simulink model "segmentCalcPos"  (R2019a)
settings: Solver=VariableStepAuto  StartTime=0  StopTime=inf  FixedStep=1e-3  MaxStep=1e-3  RelTol=1e-3
values from neighbouring files (symbols this model uses):
  apexVelocity = apexData.velocity(n,2)    [calcSegments.m]
  course = addRadius(course,max(vRLookUp(:,1)))    [calcggV.m]    (also in importCourse.m = addRadius(course))
  currentDistance = apexData.locs(n,1) - 1    [calcSegments.m]
  stoppingDistance = apexData.locs(n+1,1) - 1    [calcSegments.m]
undefined symbols (not defined in the file or in its folder): aeroMap, init
libraries: simulink x1
settings Model: Creator=Frieder Uerlings  LastModifiedBy=fried

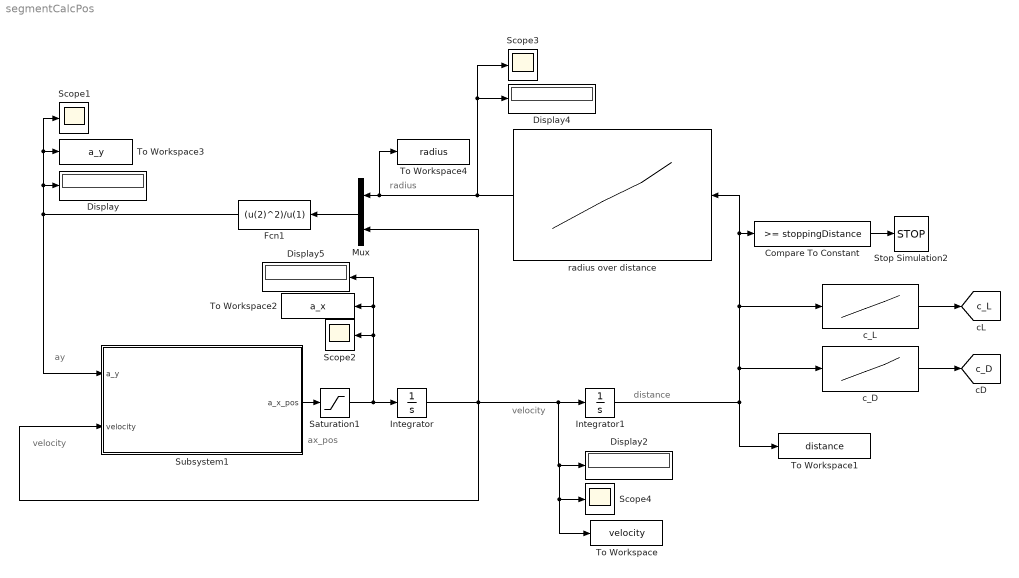
== system segmentCalcPos ==
  note: radius
  note: distance
  note: velocity
  note: velocity
  note: ay
  note: ax_pos
  Compare To Constant : simulink/Logic and Bit Operations/Compare To Constant  relop=>=  const=stoppingDistance  OutDataTypeStr=boolean
  Display{,2,4..5} (4 alike) : Display
  Fcn1 : Fcn  Expr=(u(2)^2)/u(1)
  Integrator : Integrator  InitialCondition=apexVelocity
  Integrator1 : Integrator  InitialCondition=currentDistance
  Mux : Mux  Inputs=2
  Saturation1 : Saturate  UpperLimit=inf  LowerLimit=0
  Scope{1..4} (4 alike) : Scope
  Stop Simulation2 : Stop
  Subsystem1 : Subsystem
  To Workspace : ToWorkspace  VariableName=velocity  SampleTime=-1
  To Workspace1 : ToWorkspace  VariableName=distance  SampleTime=-1
  To Workspace2 : ToWorkspace  VariableName=a_x  SampleTime=-1
  To Workspace3 : ToWorkspace  VariableName=a_y  SampleTime=-1
  To Workspace4 : ToWorkspace  VariableName=radius  SampleTime=-1
  "c_D " : Lookup_n-D  NumberOfTableDimensions=1  BreakpointsForDimension1=[0:init.ptDistance:(length(course)-1)*init.ptDistance]  Table=aeroMap(:,2)  InternalRulePriority=Speed  RndMeth=Simplest  InputSameDT=on
  c_L : Lookup_n-D  NumberOfTableDimensions=1  BreakpointsForDimension1=[0:init.ptDistance:(length(course)-1)*init.ptDistance]  Table=aeroMap(:,1)  InternalRulePriority=Speed  RndMeth=Simplest  InputSameDT=on
  radius over distance : Lookup_n-D  NumberOfTableDimensions=1  BreakpointsForDimension1=[0:init.ptDistance:(length(course)-1)*init.ptDistance]  Table=course(:,3)  InternalRulePriority=Speed  RndMeth=Simplest  InputSameDT=on
  tag scope: c_D=global, c_L=global
  wires:
  Integrator1/1 -> To Workspace1/1, "c_D "/1, c_L/1, Compare To Constant/1, radius over distance/1
  Subsystem1/1("a_x_pos ") -> Saturation1/1
  radius over distance/1 -> Scope3/1, Display4/1, To Workspace4/1, Mux/1
  Mux/1 -> Fcn1/1
  Compare To Constant/1 -> Stop Simulation2/1
  Integrator/1 -> Subsystem1/2("velocity "), Mux/2, To Workspace/1, Scope4/1, Display2/1, Integrator1/1
  Saturation1/1 -> Display5/1, To Workspace2/1, Scope2/1, Integrator/1
  Fcn1/1 -> Subsystem1/1("a_y "), Display/1, Scope1/1, To Workspace3/1
  "c_D "/1 -> [c_D]
  c_L/1 -> [c_L]

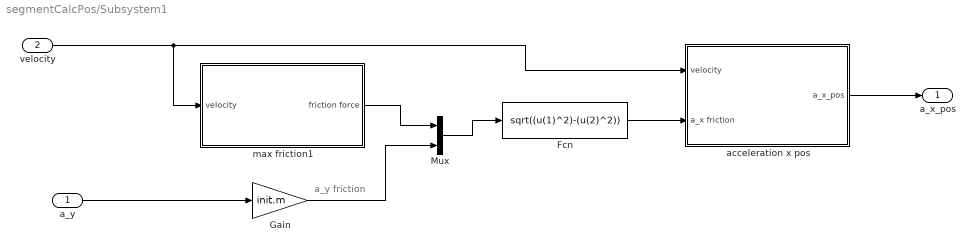
== system segmentCalcPos/Subsystem1 ==
  note: a_y friction
  "a_y " : Inport
  "velocity " : Inport  Port=2
  Fcn : Fcn  Expr=sqrt((u(1)^2)-(u(2)^2))
  Gain : Gain  Gain=init.m
  Mux : Mux  Inputs=2
  acceleration x pos : Subsystem
  max friction1 : Subsystem
  "a_x_pos " : Outport
  wires:
  "velocity "/1 -> acceleration x pos/1(velocity), max friction1/1(velocity)
  "a_y "/1 -> Gain/1
  Fcn/1 -> acceleration x pos/2(a_x friction)
  Mux/1 -> Fcn/1
  acceleration x pos/1("a_x_pos ") -> "a_x_pos "/1
  max friction1/1(friction force) -> Mux/1
  Gain/1 -> Mux/2

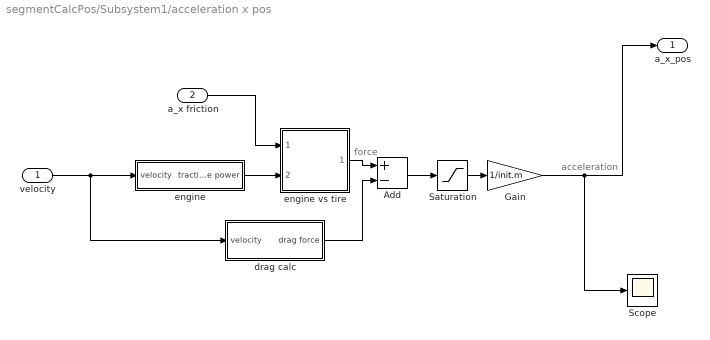
== system segmentCalcPos/Subsystem1/acceleration x pos ==
  note: force
  note: acceleration
  velocity : Inport
  a_x friction : Inport  Port=2
  Add : Sum  Inputs=+-
  Gain : Gain  Gain=1/init.m
  Saturation : Saturate  UpperLimit=inf  LowerLimit=0
  Scope : Scope
  drag calc : Subsystem
  engine : Subsystem
  engine vs tire : Subsystem
  "a_x_pos " : Outport
  wires:
  engine vs tire/1(acc force) -> Add/1
  Gain/1 -> "a_x_pos "/1, Scope/1
  Add/1 -> Saturation/1
  drag calc/1("drag force ") -> Add/2
  engine/1(tractive power) -> engine vs tire/2(tractive power)
  a_x friction/1 -> engine vs tire/1("a_x friction ")
  velocity/1 -> drag calc/1(velocity), engine/1(velocity)
  Saturation/1 -> Gain/1

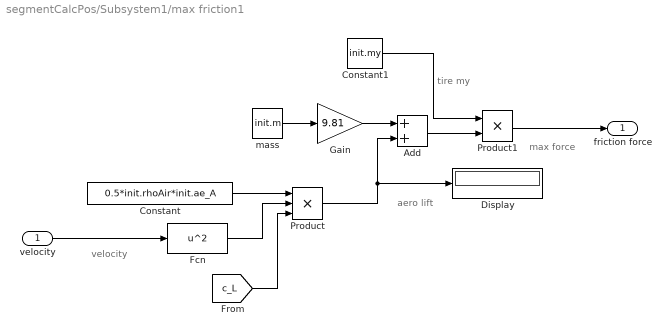
== system segmentCalcPos/Subsystem1/max friction1 ==
  note: velocity
  note: tire my
  note: aero lift
  note: max force
  velocity : Inport
  Add : Sum
  Constant : Constant  Value=0.5*init.rhoAir*init.ae_A
  Constant1 : Constant  Value=init.my
  Display : Display
  Fcn : Fcn  Expr=u^2
  Gain : Gain  Gain=9.81
  Product : Product  Inputs=3
  Product1 : Product
  "mass " : Constant  Value=init.m
  friction force : Outport
  wires:
  Product/1 -> Display/1, Add/2
  velocity/1 -> Fcn/1
  Constant1/1 -> Product1/1
  Gain/1 -> Add/1
  Product1/1 -> friction force/1
  Fcn/1 -> Product/2
  "mass "/1 -> Gain/1
  Add/1 -> Product1/2
  Constant/1 -> Product/1
  [c_L] -> Product/3

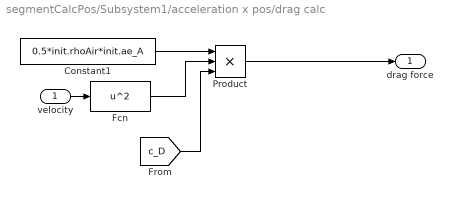
== system segmentCalcPos/Subsystem1/acceleration x pos/drag calc ==
  velocity : Inport
  Constant1 : Constant  Value=0.5*init.rhoAir*init.ae_A
  Fcn : Fcn  Expr=u^2
  Product : Product  Inputs=3
  "drag force " : Outport
  wires:
  Constant1/1 -> Product/1
  velocity/1 -> Fcn/1
  Fcn/1 -> Product/2
  Product/1 -> "drag force "/1
  [c_D] -> Product/3

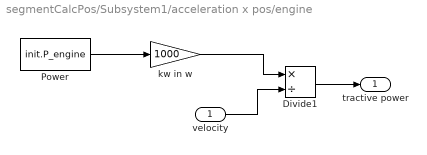
== system segmentCalcPos/Subsystem1/acceleration x pos/engine ==
  velocity : Inport
  Divide1 : Product  Inputs=*/
  "Power " : Constant  Value=init.P_engine
  "kw in w " : Gain  Gain=1000
  tractive power : Outport
  wires:
  "Power "/1 -> "kw in w "/1
  "kw in w "/1 -> Divide1/1
  Divide1/1 -> tractive power/1
  velocity/1 -> Divide1/2

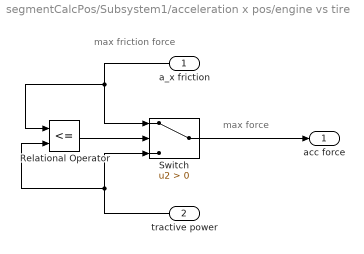
== system segmentCalcPos/Subsystem1/acceleration x pos/engine vs tire ==
  note: max force
  note: max friction force
  "a_x friction " : Inport
  tractive power : Inport  Port=2
  Relational Operator : RelationalOperator  Operator=<=  OutDataTypeStr=boolean  RndMeth=Simplest
  Switch : Switch  Criteria=u2 > Threshold
  acc force : Outport
  wires:
  tractive power/1 -> Relational Operator/2, Switch/3
  "a_x friction "/1 -> Relational Operator/1, Switch/1
  Switch/1 -> acc force/1
  Relational Operator/1 -> Switch/2
